simulink model "test05"  (Simulink 7.4)
settings: Solver=ode3  StartTime=0.0  StopTime=inf  RelTol=1e-3
undefined symbols (not defined in the file or in its folder): serial
libraries: instrumentlib x3, NAV420Lib x1
settings Model: Creator=djulzz  LastModifiedBy=djulzz
settings DebuggingCC: SolverPrmCheckMsg=none

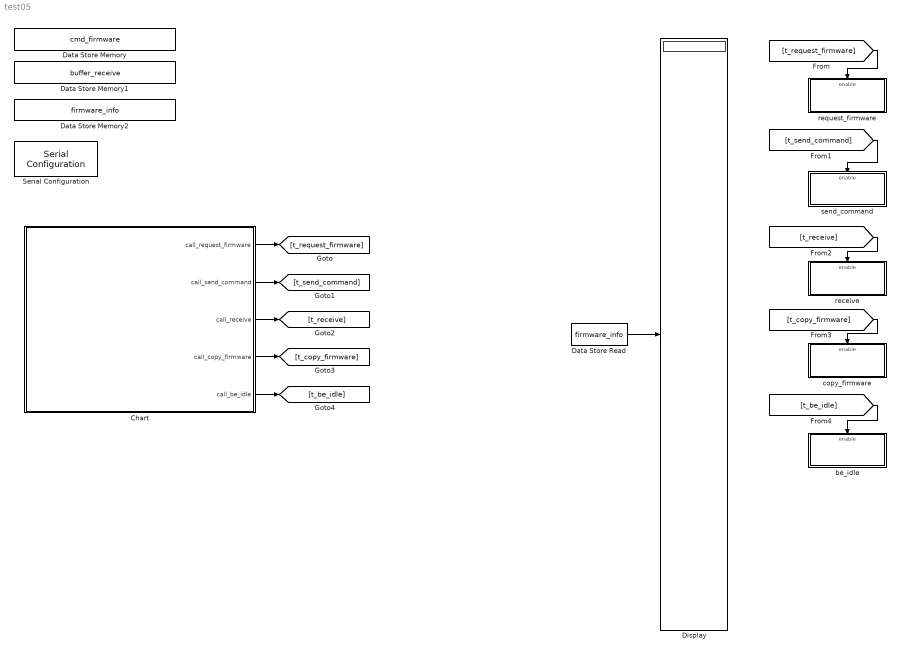
== system test05 ==
  Chart : Stateflow chart
  Data Store Memory : DataStoreMemory  DataStoreName=cmd_firmware  InitialValue=[0 0 0 0 0]  DataType=uint8  OutDataType=fixdt(1, 16)  OutScaling=2^0  OutDataTypeStr=uint8
  Data Store Memory1 : DataStoreMemory  DataStoreName=buffer_receive  InitialValue=[0; 0; 0; 0; 0; 0; 0; 0; 0; 0; 0; 0; 0; 0; 0; 0; 0; 0; 0; 0; 0; 0; 0; 0; 0; 0; 0; 0; 0; 0; 0; 0; 0; 0; 0; 0; 0; 0; 0; 0]  VectorParams1D=off  DataType=uint8  OutDataType=fixdt(1, 16)  OutScaling=2^0  OutDataTypeStr=uint8
  Data Store Memory2 : DataStoreMemory  DataStoreName=firmware_info  InitialValue=[0; 0; 0; 0; 0; 0; 0; 0; 0; 0; 0; 0; 0; 0; 0; 0; 0; 0; 0; 0; 0; 0; 0; 0; 0; 0; 0; 0; 0; 0; 0; 0; 0; 0; 0; 0; 0; 0; 0; 0]  VectorParams1D=off  DataType=uint8  OutDataType=fixdt(1, 16)  OutScaling=2^0  OutDataTypeStr=uint8
  Data Store Read : DataStoreRead  DataStoreName=firmware_info  SampleTime=-1
  Display : Display
      settings: Format=hex (Stored Integer)
  Serial Configuration : instrumentlib/Serial Configuration  Priority=-200000  DialogController=instrumentcreatedialog  DialogControllerArgs=DataTag0  ComPortMenu=COM1  ComPort=COM1  ObjConstructor=serial('COM1');  BaudRate=38400  DataBits=8  Parity=none  StopBits=1  FlowControl=none  Timeout=10  ByteOrder=LittleEndian
  be_idle : Subsystem  TreatAsAtomicUnit=on
  copy_firmware : Subsystem  TreatAsAtomicUnit=on
  receive : Subsystem  TreatAsAtomicUnit=on
  request_firmware : Subsystem  TreatAsAtomicUnit=on
  send_command : Subsystem  TreatAsAtomicUnit=on
  wires:
  [t_request_firmware] -> request_firmware/Enable
  [t_send_command] -> send_command/Enable
  [t_receive] -> receive/Enable
  [t_copy_firmware] -> copy_firmware/Enable
  [t_be_idle] -> be_idle/Enable
  Chart/5(call_be_idle) -> [t_be_idle]
  Chart/4(call_copy_firmware) -> [t_copy_firmware]
  Chart/3(call_receive) -> [t_receive]
  Chart/2(call_send_command) -> [t_send_command]
  Chart/1(call_request_firmware) -> [t_request_firmware]
  Data Store Read/1 -> Display/1

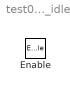
== system test05/be_idle ==
  Enable : EnablePort

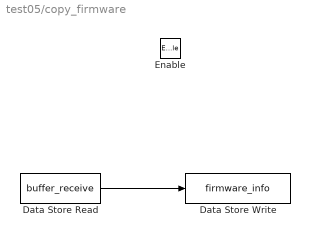
== system test05/copy_firmware ==
  Enable : EnablePort
  Data Store Read : DataStoreRead  DataStoreName=buffer_receive  SampleTime=-1
  Data Store Write : DataStoreWrite  DataStoreName=firmware_info  SampleTime=-1
  wires:
  Data Store Read/1 -> Data Store Write/1

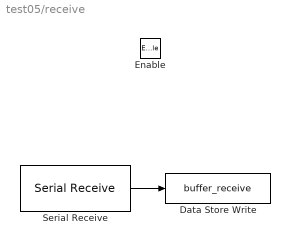
== system test05/receive ==
  Enable : EnablePort
  Data Store Write : DataStoreWrite  DataStoreName=buffer_receive  SampleTime=-1
  Serial Receive : instrumentlib/Serial Receive  DialogController=instrumentcreatedialog  DialogControllerArgs=DataTag1  ComPortMenu=COM1  ComPort=COM1  ObjConstructor=serial('COM1');  Terminator=<none>  DataSize="[40   1]"  DataType=uint8  EnableBlockingMode=on  ActionDataUnavailable=Output last received value  CustomValue=0  SampleTime=-1
  wires:
  Serial Receive/1 -> Data Store Write/1

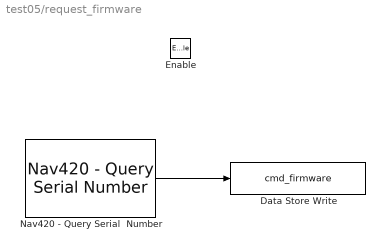
== system test05/request_firmware ==
  Enable : EnablePort
  Data Store Write : DataStoreWrite  DataStoreName=cmd_firmware  SampleTime=-1
  Nav420 - Query Serial  Number : NAV420Lib/Nav420 - Query Serial  Number  SystemSampleTime=-1
  wires:
  Nav420 - Query Serial  Number/1 -> Data Store Write/1

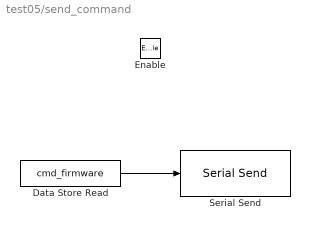
== system test05/send_command ==
  Enable : EnablePort
  Data Store Read : DataStoreRead  DataStoreName=cmd_firmware  SampleTime=-1
  Serial Send : instrumentlib/Serial Send  DialogController=instrumentcreatedialog  DialogControllerArgs=DataTag2  ComPortMenu=COM1  ComPort=COM1  ObjConstructor=serial('COM1');  Terminator=<none>  EnableBlockingMode=on
  wires:
  Data Store Read/1 -> Serial Send/1

== stateflow chart Chart ==
  state Step01
    call_request_firmware=1;
    call_send_command=1;
    call_receive=1;
    call_copy_firmware=1;
  state Step02
    call_copy_firmware=0;
    call_request_firmware=0;
    call_send_command=0;
    call_receive=0;
    call_be_idle=1;
  Step01 -> Step02 [order 1] : [firmware_info[1]==85]
  (default) -> Step01
  Step01 -> Step01 [order 2] : [firmware_info[1]~=85]
  data: cmd_firmware data_store_memory double; buffer_receive data_store_memory double; firmware_info data_store_memory double; call_request_firmware output uint8; call_send_command output uint8; call_receive output uint8; call_copy_firmware output uint8; call_be_idle output uint8
